simulink model "vexv5_Vision_Actuation"  (R2019b)
settings: Solver=FixedStepAuto  StartTime=0.0  StopTime=inf  RelTol=1e-3
libraries: vexv5lib x2, dspstat3 x2
settings Model: Creator=avenkata  LastModifiedBy=josea
settings OptimizationCC: EnhancedBackFolding=on  PassReuseOutputArgsThreshold=0  MaxStackSize=64  OptimizeBlockOrder=speed  DifferentSizesBufferReuse=on  OptimizationCustomize=off
settings DebuggingCC: ParameterTunabilityLossMsg=error  SymbolicDimsDataTypeCodeGenerationDiagnostic=none  ArithmeticOperatorsInVariantConditions=warning
settings HardwareCC: ProdBitPerPointer=32  ProdBitPerSizeT=32  ProdBitPerPtrDiffT=32  ProdLargestAtomicInteger=Long  ProdLargestAtomicFloat=Double  ProdWordSize=32  ProdHWDeviceType=ARM Compatible->ARM Cortex  UseEmbeddedCoderFeatures=off
settings SFSimCC: MATLABDynamicMemAlloc=off  CustomCodeUndefinedFunction=UseInterfaceOnly
settings RTWCC: SystemTargetFile=ert.tlc  HardwareBoard=VEX V5 Robot Brain  TLCOptions="-aInlineSetEventsForThisBaseRateFcn=TLC_FALSE -aSuppressMultiTaskScheduler=TLC_FALSE  -aRateBasedStepFcn=0"  TemplateMakefile=ert_default_tmf  GenerateReport=on  Toolchain=GNU Tools for ARM Embedded Processors  LaunchReport=on
settings CodeAppCC: ForceParamTrailComments=on  OperatorAnnotations=on
settings ERTTargetCC: ERTCustomFileBanners=off  SupportContinuousTime=on  SupportNonInlinedSFcns=on  RemoveResetFunc=off  ModelStepFunctionPrototypeControlCompliant=off

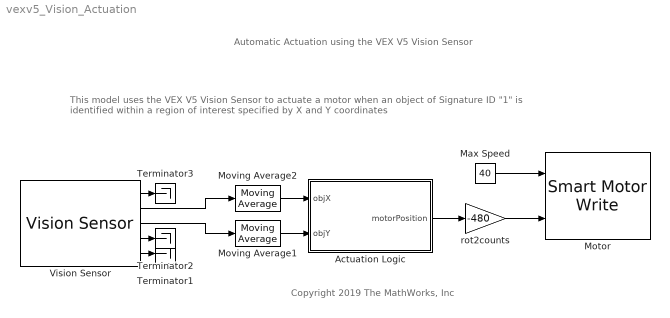
== system vexv5_Vision_Actuation ==
  note: This model uses the VEX V5 Vision Sensor to actuate a motor when an object of Signature ID "1"
      | is identified within a region of interest specified by X and Y coordinates
  note: Automatic Actuation
      | using the VEX V5 Vision Sensor
  note: Copyright 2019 The MathWorks, Inc
  Actuation Logic : Stateflow chart  TreatAsAtomicUnit=on
  Max Speed : Constant  Value=40
  Motor : vexv5lib/Actuators/Smart Motor Write  motorPort=3  scaleFactor=18:1  MotorBrakeMode=Hold  OperationMode=Position Control
      settings: SourceProductName=Simulink Coder Support Package for VEX EDR V5 Robot Brain
  Moving Average1 : dspstat3/Moving Average  Method=Sliding window  ForgettingFactorPort=off  SpecifyWindowLength=on  WindowLength=4  ForgettingFactor=0.9  SimulateUsing=Code generation
  Moving Average2 : dspstat3/Moving Average  Method=Sliding window  ForgettingFactorPort=off  SpecifyWindowLength=on  WindowLength=4  ForgettingFactor=0.9  SimulateUsing=Code generation
  Terminator1 : Terminator
  Terminator2 : Terminator
  Terminator3 : Terminator
  Vision Sensor : vexv5lib/Sensors/Vision Sensor  Port=5  EnableColorCode=off  ColorCode=12  SigId=SIG_1  size=1  LCDOutput=on  SampleTime=0.2
      settings: SourceProductName=Simulink Coder Support Package for VEX EDR V5 Robot Brain  SourceProductBaseCode=VEXV5
  rot2counts : Gain  Gain=-480
  wires:
  Vision Sensor/2 -> Moving Average2/1
  Vision Sensor/3 -> Moving Average1/1
  Moving Average2/1 -> Actuation Logic/1(objX)
  Moving Average1/1 -> Actuation Logic/2(objY)
  Max Speed/1 -> Motor/1
  Actuation Logic/1(motorPosition) -> rot2counts/1
  rot2counts/1 -> Motor/2
  Vision Sensor/4 -> Terminator2/1
  Vision Sensor/5 -> Terminator1/1
  Vision Sensor/1 -> Terminator3/1

== stateflow chart vexv5_Vision_Actuation/Actuation Logic ==
  state Idle
    motorPosition=1;
  state Release
    motorPosition=1;
  state Grab
    motorPosition=0;
  (default) -> Idle
  Release -> Idle : after(3,sec)
  Idle -> Grab : [objX > 170 && objX < 200 &&...
      | objY > 170 && objY < 195]
  Grab -> Release : after(5,sec)
  data: motorPosition output; objX input; objY input
